simulink model "practical_class_3_1c_simulink"  (R2023b)
settings: Solver=VariableStepAuto  StartTime=0.0  StopTime=8  RelTol=1e-3
values from neighbouring files (symbols this model uses):
  A = [0, -1/L; 1/C, -1/(R*C)]    [practical_class_3_1c.m]
  B = [1/L; 0]    [practical_class_3_1c.m]
  c2 = [0 -1]    [practical_class_3_1c.m]
  D2 = 1    [practical_class_3_1c.m]
settings Model: Creator=klysm  LastModifiedBy=klysm

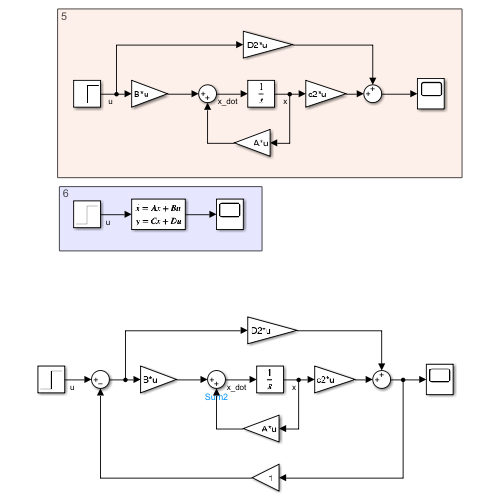
[thumbnail: Simulink's stored preview of the top-level diagram]
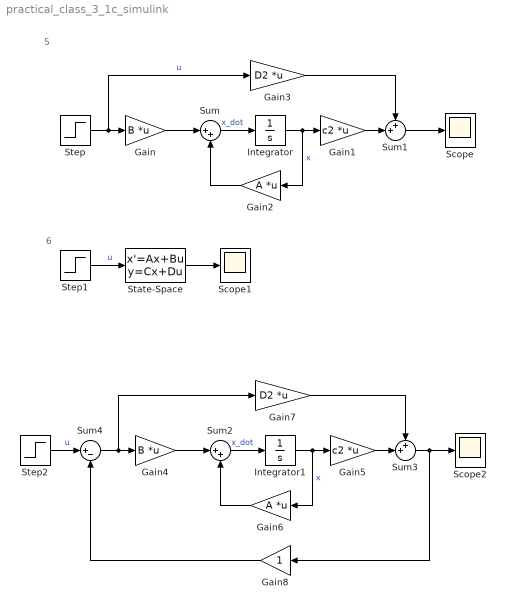
== system practical_class_3_1c_simulink ==
  note: 6
  note: 5
  Gain : Gain  Gain=B  Multiplication=Matrix(K*u)
  Gain1 : Gain  Gain=c2  Multiplication=Matrix(K*u)
  Gain2 : Gain  Gain=A  Multiplication=Matrix(K*u)
  Gain3 : Gain  Gain=D2  Multiplication=Matrix(K*u)
  Gain4 : Gain  Gain=B  Multiplication=Matrix(K*u)
  Gain5 : Gain  Gain=c2  Multiplication=Matrix(K*u)
  Gain6 : Gain  Gain=A  Multiplication=Matrix(K*u)
  Gain7 : Gain  Gain=D2  Multiplication=Matrix(K*u)
  Gain8 : Gain
  Integrator : Integrator
  Integrator1 : Integrator
  Scope : Scope
  Scope1 : Scope
  Scope2 : Scope
  State-Space : StateSpace  A=A  B=B  C=c2  D=D2  InitialCondition=0
  Step : Step  Time=0  SampleTime=0
  Step1 : Step  Time=0  SampleTime=0
  Step2 : Step  Time=0  SampleTime=0
  Sum : Sum  Inputs=|++
  Sum1 : Sum  Inputs=++|
  Sum2 : Sum  Inputs=|++
  Sum3 : Sum  Inputs=++|
  Sum4 : Sum  Inputs=|+-
  wires:
  Step/1 -> Gain3/1, Gain/1  "u"
  Gain/1 -> Sum/1
  Sum/1 -> Integrator/1  "x_dot"
  Integrator/1 -> Gain2/1, Gain1/1  "x"
  Gain1/1 -> Sum1/2
  Gain2/1 -> Sum/2
  Gain3/1 -> Sum1/1
  Step1/1 -> State-Space/1  "u"
  State-Space/1 -> Scope1/1
  Sum1/1 -> Scope/1
  Gain6/1 -> Sum2/2
  Sum2/1 -> Integrator1/1  "x_dot"
  Sum4/1 -> Gain7/1, Gain4/1
  Integrator1/1 -> Gain6/1, Gain5/1  "x"
  Gain7/1 -> Sum3/1
  Gain5/1 -> Sum3/2
  Sum3/1 -> Gain8/1, Scope2/1
  Gain4/1 -> Sum2/1
  Step2/1 -> Sum4/1  "u"
  Gain8/1 -> Sum4/2
